simulink model "cruiseco"  (R2020b)
settings: Solver=ode45  StartTime=0.0  StopTime=120  RelTol=1e-3
model workspace (MAT data in the model file):
  b = 50
  kd = 300
  ki = 50
  kp = 350
  m = 1000
  meViews.Name = 'Dictionary Objects'
  meViews.Domain = 'Simulink'
  meViews.Description = 'Show common properties for data objects and variables in dictionaries'
  meViews.InternalName = 'TMW_Dictionary Objects_SimulinkCoderNotAvailable'
  meViews.GroupName = ''
  meViews.SortName = ''
  meViews.SortOrder = ''
  meViews.Properties : DAStudio.MEViewProperty (value not decoded)
  u = 500
settings Model: Creator=com  LastModifiedBy=com

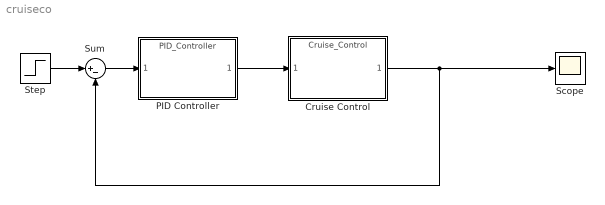
== system cruiseco ==
  Cruise Control : ModelReference  ModelNameDialog=Cruise_Control  ModelReferenceVersion=1.3
  PID Controller : ModelReference  ModelNameDialog=PID_Controller  ModelReferenceVersion=1.3
  Scope : Scope
  Step : Step  After=u  SampleTime=0
  Sum : Sum  Inputs=|+-
  wires:
  Cruise Control/1 -> Sum/2, Scope/1
  PID Controller/1 -> Cruise Control/1
  Sum/1 -> PID Controller/1
  Step/1 -> Sum/1
